simulink model "three_c_attitude_control_quaternion"  (R2021a)
settings: Solver=ode23t  StartTime=0.0  StopTime=100  RelTol=1e-5
undefined symbols (not defined in the file): g, I, km, kt, L, m, pm_0, q_init, sigbuilder_block, thrust_max, TQ_max_per_motor, Vb_init, Vm_0, wb_init, Xe_init, xme_0
libraries: simulink_extras x18, aerolibutil x4, sharedtransform x2, simulink x2, sharedutil x1
(part 2 of 2)

== matlab function three_c_attitude_control_quaternion/Control allocation and motor control/Ideal Actuators with allocation/Control allocation/FM_to_w2 ==
  data: L input; w2_cmd output; kt input; km input; Thrust input; M_x input; M_y input; M_z input
function w2_cmd = control_allocation(L, kt, km, Thrust, M_x, M_y, M_z)
%#codegen

    % construct the co-efficient matrix:
    %  F_and_M = C * w^2
    %
    % C = [
    %     kt  ,   kt   ,   kt  ,   kt  ;
    %     0   , -L*kt  ,   0   , L*kt  ;
    %    L*kt ,   0    , -L*kt ,   0   ;
    %     km ,   -km   ,  km  ,   -km  ;
    % ];

    % used Symbolic toolbox to compute inv(C)
%     C_inv = [
%                 1/(4*kt),          0 ,  1/(2*L*kt),  1/(4*km);
%                 1/(4*kt), -1/(2*L*kt),           0,  -1/(4*km); 
%                 1/(4*kt),          0 , -1/(2*L*kt),  1/(4*km);
%                 1/(4*kt), 1/(2*L*kt) ,          0 ,  -1/(4*km);
%              ];
         
    C_inv = [
             -1/(4*kt),            0,   1/(2*L*kt), -1/(4*km);
             -1/(4*kt),  -1/(2*L*kt),            0,  1/(4*km);
             -1/(4*kt),            0,  -1/(2*L*kt), -1/(4*km);
             -1/(4*kt),   1/(2*L*kt),            0,  1/(4*km);
            ];        
    % solve for the w^2 vec
    F_and_M_col = [Thrust, M_x, M_y, M_z].' ;

    w2_cmd = C_inv * F_and_M_col;
   
end

== matlab function three_c_attitude_control_quaternion/Quad_EOM/Integrate_quaternion/Calc Euler_rates/euler_rates ==
  data: phi_t input; euler_rates output; theta_t input; p input; q input; r input
function euler_rates = euler_rates(phi_t,theta_t,p,q,r)
%#codegen

%    This function was generated by the Symbolic Math Toolbox version 8.7.
%    04-Nov-2022 08:55:55

euler_rates = [(p.*cos(theta_t)+r.*cos(phi_t).*sin(theta_t)+q.*sin(phi_t).*sin(theta_t))./cos(theta_t);q.*cos(phi_t)-r.*sin(phi_t);(r.*cos(phi_t)+q.*sin(phi_t))./cos(theta_t)];

== matlab function three_c_attitude_control_quaternion/Quad_EOM/Integrate_quaternion/MATLAB Function2 ==
  data: R input; phi output; theta output; psi output
function [phi,theta,psi] = euler_from_rot(R)
% Get Euler angles from rotation matrix (wolrd to body rotation matrix)
%NOTE:  this is bRg ... and NOT gRb

phi   = atan2(R(2,3),R(3,3));
theta = -asin(R(1,3));
psi   = atan2(R(1,2), R(1,1));
end

== matlab function three_c_attitude_control_quaternion/Control allocation and motor control/Ideal Actuators with allocation/Perfect actuators/Allocation matrix (motor speed to twist) ==
  data: L input; Thrust output; kt input; km input; w2_col input; M_x output; M_y output; M_z output
function [Thrust, M_x, M_y, M_z] = mixer(L, kt, km, w2_col)
%#codegen



    % construct the co-efficient matrix:
    %  T = C * w^2
    
%     C = [
%         kt  ,   kt   ,   kt  ,   kt  ;
%         0   , -L*kt  ,   0   , L*kt  ;
%        L*kt ,   0    , -L*kt ,   0   ;
%         km ,   -km   ,  km  ,   -km  ;
%     ];

    C = [
        -kt  ,   -kt  ,   -kt ,   -kt  ;
        0    , -L*kt   ,   0   , L*kt  ;
       L*kt ,   0    , -L*kt  ,   0   ;
        -km  ,   km   ,  -km  ,   km  ;
    ];

    % solve for the FM_col
    %   FM_col = [Thrust, M_x, M_y, M_z].' ;
    
    FM_col  =  C * w2_col;
    
    Thrust  =  FM_col(1);
    M_x     =  FM_col(2);
    M_y     =  FM_col(3);
    M_z     =  FM_col(4);
    
end

== matlab function three_c_attitude_control_quaternion/Quad_EOM/Integrate_quaternion/calc_bRg ==
  data: q input double size=[4, 1]; bRg output double size=[3 3]
function bRg = quat2dcm(q)
% convert quaternion to DCM
% the DCM represent coordinate transformation of a vector in inertial axes
% into body axes (bRg)

% VERY SLOW in SIMULINK

    q0    = q(1);
    qx    = q(2);
    qy    = q(3);
    qz    = q(4);
    
    C_11  = qx^2 + q0^2 - qy^2 - qz^2;
    C_12  = 2*(qx*qy + qz*q0);
    C_13  = 2*(qx*qz - qy*q0);
       
    C_21  = 2*(qx*qy - qz*q0);
    C_22  = qy^2 + q0^2 - qx^2 - qz^2;
    C_23  = 2*(qy*qz + qx*q0);
    
    C_31  = 2*(qx*qz + qy*q0);
    C_32  = 2*(qy*qz - qx*q0);
    C_33  = qz^2 + q0^2 - qx^2 - qy^2;
    
    
    bRg = [ C_11, C_12, C_13;
            C_21, C_22, C_23;
            C_31, C_32, C_33;   ];   


end

== matlab function three_c_attitude_control_quaternion/Quad_EOM/Integrate_quaternion/calc_q_DOT ==
  data: q input double size=[4, 1]; q_dot output double size=[4 1]; wb input double size=[3, 1]
function q_dot = q_dot_from_rates(q, wb)
% angular rates are related to quaternion derivative by:
% note: this transformation is in body-fixed frame (body rates and
% quaternion in body-fixed frame)
% q_dot  = 0.5 * W^T * wb;
% 
% W = 
%    [-q1,  q0,  q3, -q2]
%    [-q2, -q3,  q0,  q1]
%    [-q3,  q2, -q1,  q0]
% W_transpose = 
%             [-q1, -q2, -q3]
%             [ q0, -q3,  q2]
%             [ q3,  q0, -q1]
%             [-q2,  q1,  q0]

q0     = q(1);
q1     = q(2);
q2     = q(3);
q3     = q(4);

W_transpose =  [
                 -q1, -q2, -q3;
                  q0, -q3,  q2;
                  q3,  q0, -q1;
                 -q2,  q1,  q0;
                 ];

wb = wb(:);

q_dot  = 0.5 * W_transpose * wb;

end
